simulink model "psd_reg"  (R2024b)
settings: Solver=VariableStepAuto  StartTime=tspan(1)  StopTime=tspan(2)  RelTol=1e-3
values from neighbouring files (symbols this model uses):
  dtflin = dtftust(tflin, Ts)    [disc.m]    (also in main.m)
  PSDMomReg = PSD(MomReg, Ts)    [main.m]
  PSDNaslinReg = PSD(NaslinReg, Ts_reg)    [main.m]
  z = -0.1    [main.m]
settings Model: Creator=markminerov  LastModifiedBy=markminerov
settings DebuggingCC: AlgebraicLoopMsg=none

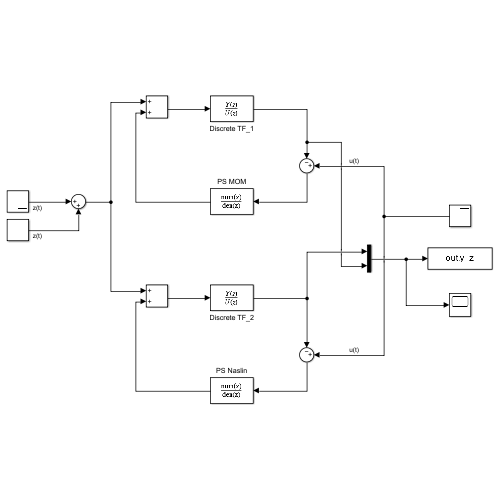
[thumbnail: Simulink's stored preview of the top-level diagram]
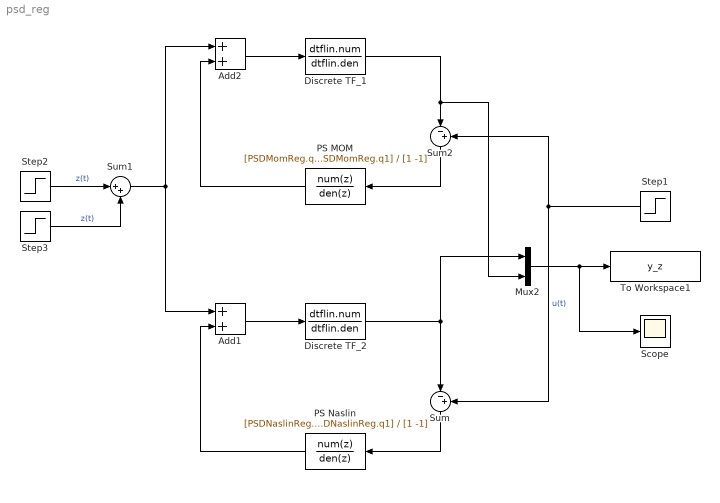
== system psd_reg ==
  Add1 : Sum
  Add2 : Sum
  Discrete TF_1 : DiscreteTransferFcn  Numerator=dtflin.num  Denominator=dtflin.den
  Discrete TF_2 : DiscreteTransferFcn  Numerator=dtflin.num  Denominator=dtflin.den
  Mux2 : Mux  Inputs=2
  PS MOM : DiscreteTransferFcn  Numerator=[PSDMomReg.q0 PSDMomReg.q1]  Denominator=[1 -1]
  PS Naslin : DiscreteTransferFcn  Numerator=[PSDNaslinReg.q0 PSDNaslinReg.q1]  Denominator=[1 -1]
  Scope : Scope
  Step1 : Step  After=u  SampleTime=0
  Step2 : Step  Time=11  After=z  SampleTime=0
  Step3 : Step  Time=12  After=-z  SampleTime=0
  Sum : Sum  Inputs=|-+
  Sum1 : Sum  Inputs=|++
  Sum2 : Sum  Inputs=|-+
  To Workspace1 : ToWorkspace  VariableName=y_z  SaveFormat=Timeseries  SampleTime=-1
  wires:
  Sum1/1 -> Add2/1, Add1/1
  Discrete TF_2/1 -> Mux2/1, Sum/1
  Sum/1 -> PS Naslin/1
  Add1/1 -> Discrete TF_2/1
  PS Naslin/1 -> Add1/2
  Step2/1 -> Sum1/1  "z(t)"
  Step3/1 -> Sum1/2  "z(t)"
  Mux2/1 -> Scope/1, To Workspace1/1
  PS MOM/1 -> Add2/2
  Discrete TF_1/1 -> Mux2/2, Sum2/1
  Sum2/1 -> PS MOM/1
  Step1/1 -> Sum/2, Sum2/2  "u(t)"
  Add2/1 -> Discrete TF_1/1
